simulink model "example_model_demo"  (R2015b)
settings: Solver=ode4  StartTime=0.0  StopTime=10.0  FixedStep=1e-3  RelTol=1e-3
undefined symbols (not defined in the file): params, x1_ic
settings Model: Creator=reiter  LastModifiedBy=reiter
settings ConfigComp: CovModelRefEnable=Off

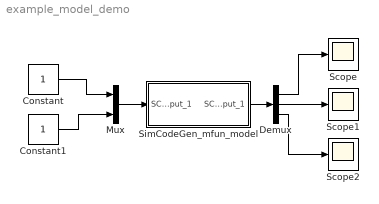
== system example_model_demo ==
  Constant : Constant
  Constant1 : Constant
  Demux : Demux  Outputs=3
  Mux : Mux  Inputs=2
  Scope : Scope
  Scope1 : Scope
  Scope2 : Scope
  SimCodeGen_mfun_model : Subsystem  mask{SC_param_0=params, SC_x1_ic=x1_ic}
      mask prompts: SC_param_0 "params"
      mask Display:
      | port_label('input', 1, 'u');
      | port_label('output', 1, 'h');
  wires:
  Mux/1 -> SimCodeGen_mfun_model/1(SC_input_1)
  SimCodeGen_mfun_model/1(SC_output_1) -> Demux/1
  Constant1/1 -> Mux/2
  Constant/1 -> Mux/1
  Demux/1 -> Scope/1
  Demux/2 -> Scope1/1
  Demux/3 -> Scope2/1

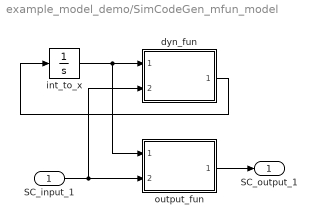
== system example_model_demo/SimCodeGen_mfun_model ==
  SC_input_1 : Inport
  dyn_fun : MATLAB Function  TreatAsAtomicUnit=on
  int_to_x : Integrator  InitialCondition=[SC_x1_ic]
  output_fun : MATLAB Function  TreatAsAtomicUnit=on
  SC_output_1 : Outport
  wires:
  SC_input_1/1 -> dyn_fun/2(SC_input_0), output_fun/2(SC_input_0)
  int_to_x/1 -> output_fun/1(SC_state), dyn_fun/1(SC_state)
  output_fun/1(SC_output_0) -> SC_output_1/1
  dyn_fun/1(SC_state_dot) -> int_to_x/1

== matlab function example_model_demo/SimCodeGen_mfun_model/output_fun ==
  data: SC_state input size=[3]; SC_output_0 output size=[3]; SC_input_0 input size=[2]; SC_param_0 parameter size=[2]
function SC_output_0  = y_fun(SC_state, SC_input_0, SC_param_0)
    SC_output_0 = zeros(3,1);
    SC_state_x_0 = SC_state(1:3);
    SC_output_0(1) = SC_state_x_0(1);
    SC_output_0(2) = SC_state_x_0(2);
    SC_output_0(3) = SC_state_x_0(3) * SC_input_0(1) * SC_input_0(2);
end

== matlab function example_model_demo/SimCodeGen_mfun_model/dyn_fun ==
  data: SC_state input size=[3]; SC_state_dot output size=[3]; SC_input_0 input size=[2]; SC_param_0 parameter
function SC_state_dot  = dyn_fun(SC_state, SC_input_0, SC_param_0)
    SC_state_dot = zeros(3, 1);
    SC_state_x_0 = SC_state(1:3);
    SC_eval = zeros(3,1);
    SC_eval(1) = SC_state_x_0(2);
    SC_eval(2) = -SC_param_0(2) * SC_eval(1) - SC_param_0(1) * SC_state_x_0(1) + SC_input_0(1);
    SC_eval(3) = -0.12e0 * SC_state_x_0(3);
    SC_state_dot(1:3) = SC_eval(1:3);
end
